simulink model "mas_sim_loopshaping"  (R2016b)
settings: Solver=ode45  StartTime=0.0  StopTime=300  RelTol=1e-3  EnableMultiTasking=on
InitFcn:
  | param
undefined symbols (not defined in the file or in its folder): drawMassSys, mass_ctrl_loop, P
settings Model: Creator=beard  LastModifiedBy=Jacob
settings DataIOCC: LimitDataPoints=on  SaveFormat=Array  SignalLoggingSaveFormat=ModelDataLogs
settings OptimizationCC: ExpressionDepthLimit=2147483647  InitFltsAndDblsToZero=on  LifeSpan=inf
settings DebuggingCC: UnderspecifiedInitializationDetection=Classic  MergeDetectMultiDrivingBlocksExec=none  SolverPrmCheckMsg=warning  FcnCallInpInsideContextMsg=warning  StateNameClashWarn=warning  SFUnexpectedBacktrackingDiag=warning  SFNoUnconditionalDefaultTransitionDiag=warning  SFExecutionAtInitializationDiag=none
settings HardwareCC: ProdBitPerPointer=32  ProdBitPerSizeT=32  ProdBitPerPtrDiffT=32  ProdLargestAtomicFloat=None  ProdIntDivRoundTo=Undefined  ProdEndianess=Unspecified  ProdWordSize=32  ProdHWDeviceType=32-bit Generic
settings ModelReferenceCC: PropagateSignalLabelsOutOfModel=off
settings GRTTargetCC: TargetLangStandard=C89/C90 (ANSI)  GeneratePreprocessorConditionals=Disable all  CombineOutputUpdateFcns=off  GRTInterface=on
settings ConfigComp: CovMetricSettings=dw  CovHtmlReporting=on  CovSaveCumulativeToWorkspaceVar=on  CovSaveSingleToWorkspaceVar=on  CovExternalEMLEnable=off

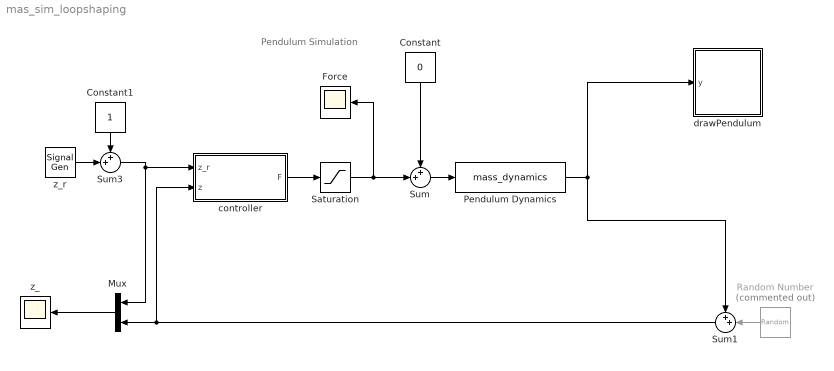
== system mas_sim_loopshaping ==
  note: Pendulum Simulation
  Constant : Constant  Value=0
  Constant1 : Constant
  Force : Scope
  Mux : Mux  Inputs=2
  Pendulum Dynamics : S-Function  FunctionName=mass_dynamics  Parameters=P  SFunctionDeploymentMode=off  EnableBusSupport=off
  Random Number : RandomNumber  Commented=on  Variance=.001^2  SampleTime=P.Ts
  Saturation : Saturate  UpperLimit=5  LowerLimit=-5
  Sum : Sum  Inputs=++|
  Sum1 : Sum  Inputs=++|
  Sum3 : Sum  Inputs=++|
  controller : Subsystem
  drawPendulum : Subsystem
      mask Display: image(imread('tv.jpg'))
  z_ : Scope
  z_r : SignalGenerator  WaveForm=square  Amplitude=.5  Frequency=.04
  wires:
  Pendulum Dynamics/1 -> Sum1/1, drawPendulum/1(y)
  controller/1(F) -> Saturation/1
  Saturation/1 -> Sum/2, Force/1
  Mux/1 -> z_/1
  Sum/1 -> Pendulum Dynamics/1
  Sum1/1 -> controller/2(z), Mux/2
  Random Number/1 -> Sum1/2
  Constant/1 -> Sum/1
  z_r/1 -> Sum3/2
  Sum3/1 -> Mux/1, controller/1(z_r)
  Constant1/1 -> Sum3/1

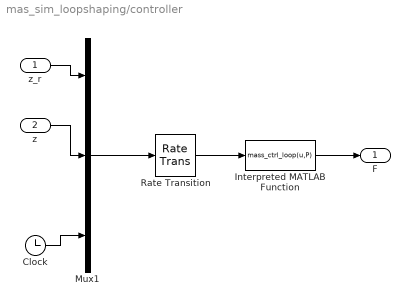
== system mas_sim_loopshaping/controller ==
  z_r : Inport
  z : Inport  Port=2
  Clock : Clock
  Interpreted MATLAB Function : MATLABFcn  MATLABFcn=mass_ctrl_loop(u,P)  OutputDimensions=1
  Mux1 : Mux  Inputs=3
  Rate Transition : RateTransition  OutPortSampleTime=P.Ts
  F : Outport
  wires:
  Mux1/1 -> Rate Transition/1
  z_r/1 -> Mux1/1
  Rate Transition/1 -> Interpreted MATLAB Function/1
  z/1 -> Mux1/2
  Interpreted MATLAB Function/1 -> F/1
  Clock/1 -> Mux1/3

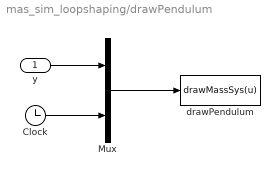
== system mas_sim_loopshaping/drawPendulum ==
  y : Inport
  Clock : Clock
  Mux : Mux  Inputs=2
  drawPendulum : MATLABFcn  MATLABFcn=drawMassSys(u)  OutputDimensions=0  SampleTime=0.1
  wires:
  Mux/1 -> drawPendulum/1
  y/1 -> Mux/1
  Clock/1 -> Mux/2
